simulink model "dft_bank_2"  (Simulink 7.8)
settings: Solver=ode45  StartTime=0.0  StopTime=1  RelTol=1e-3
values from neighbouring files (symbols this model uses):
  N = 2    [CFIR_1.m]    (also in TP_fdesign2.m = 128; cic_dezim1.m = ',num2str(N),')']); cic_dezim1_.m = ', num2str(N),' Gain = ',num2str(Hm.gain)]); cic_dezim2.m = ',num2str(N),')']))
  Ts = 1/fs    (= 6.25e-05)    [G722_1.m]    (also in adaptiv_2.m = 0.001; adaptiv_3.m = 0.001; adaptiv_4.m = 0.001; adaptiv_5.m = 0.001)
undefined symbols (not defined in the file or in its folder): Fs, get, sided, Two, WN
libraries: dspobslib x2, dspbuff3 x1, simulink x1, dspsnks4 x1
settings Model: Creator=svenhoffmann  LastModifiedBy=josef  ExtModeAutoUpdateStatusClock=off
settings DataIOCC: SignalLoggingName=sigsOut
settings OptimizationCC: InitFltsAndDblsToZero=on
settings DebuggingCC: SaveWithParameterizedLinksMsg=none  SignalResolutionControl=TryResolveAllWithWarning  SolverPrmCheckMsg=none  MultiTaskDSMMsg=warning  MultiTaskCondExecSysMsg=none  FcnCallInpInsideContextMsg=Use local settings  StrictBusMsg=None
settings HardwareCC: TargetUnknown=on
settings RTWCC: IncludeERTFirstTime=on
settings GRTTargetCC: TargetFcnLib=ansi_tfl_tmw.mat

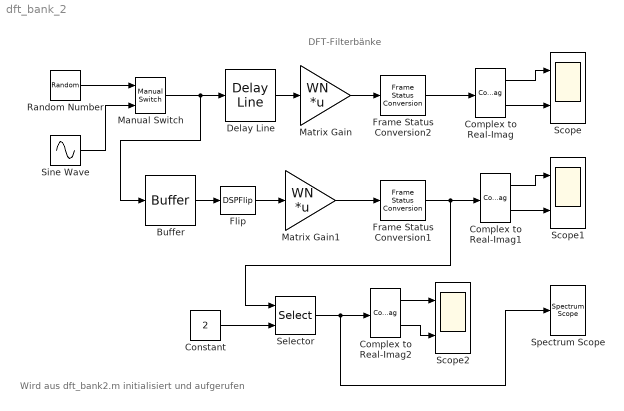
== system dft_bank_2 ==
  note: DFT-Filterbänke
  note: Wird aus dft_bank2.m initialisiert und
      | aufgerufen
  Buffer : Buffer  N=N  V=N-1
  Complex to Real-Imag : ComplexToRealImag
  Complex to Real-Imag1 : ComplexToRealImag
  Complex to Real-Imag2 : ComplexToRealImag
  Constant : Constant  Value=2
  Delay Line : dspbuff3/Delay Line  siz=N  ic=0  directfeed=off  enable_output=off  hold_output=off  TreatMby1Signals=M channels (this choice will be removed - see release notes)
  Flip : DSPFlip
  Frame Status Conversion1 : dspobslib/Frame Status Conversion  growRefPort=off  outframe=Sample-based
  Frame Status Conversion2 : dspobslib/Frame Status Conversion  growRefPort=off  outframe=Sample-based
  Manual Switch : simulink/Signal Routing/Manual Switch  sw=0  action=0  varsize=off
  Matrix Gain : Gain  Gain=WN  Multiplication=Matrix(K*u)  SaturateOnIntegerOverflow=on  OutDataTypeStr=Inherit: Same as input  ParamDataTypeStr=Inherit: Same as input
  Matrix Gain1 : Gain  Gain=WN  Multiplication=Matrix(K*u)  SaturateOnIntegerOverflow=on  OutDataTypeStr=Inherit: Same as input  ParamDataTypeStr=Inherit: Same as input
  Random Number : RandomNumber  SampleTime=Ts
  Scope : Scope  NumInputPorts=2
      settings: TimeRange=0.2  YMin=-5~-5  YMax=5~5
  Scope1 : Scope  NumInputPorts=2
      settings: TimeRange=0.2  YMin=-5~-5  YMax=5~5
  Scope2 : Scope  NumInputPorts=2
      settings: TimeRange=0.2  YMin=-5~-5  YMax=5~5  SaveName=ScopeData2
  Selector : Selector  InputPortWidth=10  IndexOptions=Index vector (port)  Indices=[2]  OutputSizes=1
  Sine Wave : Sin  Frequency=2*pi*100  Phase=pi/3  SampleTime=Ts
  Spectrum Scope : dspsnks4/Spectrum Scope  ScopeProperties=off  Domain=Frequency  HorizSpan=1  UseBuffer=on  BufferSize=256  Overlap=0  TreatMby1Signals=M channels  inpFftLenInherit=off  FFTlength=128  numAvg=5  DisplayProperties=off  AxisGrid=on  Memory=off  FrameNumber=on  AxisLegend=off  AxisZoom=off  OpenScopeAtSimStart=on  OpenScopeImmediately=off  FigPos=get(0,'defaultfigureposition')  AxisProperties=on  XUnits=Hertz  XRange=Two-sided ((-Fs/2...Fs/2])  XDisplay=0  InheritXIncr=on  XIncr=1.0  XLabel=Samples  XLimit=Auto  YUnits=dBW/Hertz  XMax=1  XMin=0  YLabel=Magnitude, dB  LineProperties=off  wintypeSpecScope=Hann  RsSpecScope=50  betaSpecScope=5  winsampSpecScope=Periodic  XAxisParamsVer=6.8  isFrameUpgraded=on
      settings: YMin=-83.7625181898217  YMax=16.024190623206
  wires:
  Random Number/1 -> Manual Switch/1
  Sine Wave/1 -> Manual Switch/2
  Manual Switch/1 -> Delay Line/1, Buffer/1
  Delay Line/1 -> Matrix Gain/1
  Buffer/1 -> Flip/1
  Flip/1 -> Matrix Gain1/1
  Matrix Gain1/1 -> Frame Status Conversion1/1
  Matrix Gain/1 -> Frame Status Conversion2/1
  Complex to Real-Imag/2 -> Scope/2
  Frame Status Conversion2/1 -> Complex to Real-Imag/1
  Complex to Real-Imag/1 -> Scope/1
  Frame Status Conversion1/1 -> Complex to Real-Imag1/1, Selector/1
  Complex to Real-Imag1/1 -> Scope1/1
  Complex to Real-Imag1/2 -> Scope1/2
  Constant/1 -> Selector/2
  Complex to Real-Imag2/1 -> Scope2/1
  Complex to Real-Imag2/2 -> Scope2/2
  Selector/1 -> Complex to Real-Imag2/1, Spectrum Scope/1
